simulink model "simul3"  (R2023b)
settings: Solver=ode4  StartTime=0.0  StopTime=600  FixedStep=0.0002  RelTol=1e-3
InitFcn:
  | init3
StopFcn:
  | stop3
values from neighbouring files (symbols this model uses):
  eps_capteur = +0.03    (= 0.03)    [init3.m]
  fs = 5000    [init3.m]
  G_pga = G_pga_vib    (= 10)    [init3.m]
  G_pga_choc = Vref_adc / (plage_g_choc * K_s)    (= 1)    [init3.m]
  G_pga_vib = Vref_adc / (plage_g_vib  * K_s)    (= 10)    [init3.m]
  K_s = 50e-3    (= 0.05)    [init3.m]
  LSB_V = 2 * Vref_adc / 2^n_bits    (= 0.000152587890625)    [init3.m]
  M_dec = 10    [init3.m]
  ordre_aaf = 4    [init3.m]
  tau_IEPE = 1 / (2 * pi * f_c_IEPE)    (= 0.318309886184)    [init3.m]
libraries: dspfdesign x1, simulink x1, dspmlti4 x1
settings Model: Creator=xavie  LastModifiedBy=xavie
settings DataIOCC: ReturnWorkspaceOutputs=off

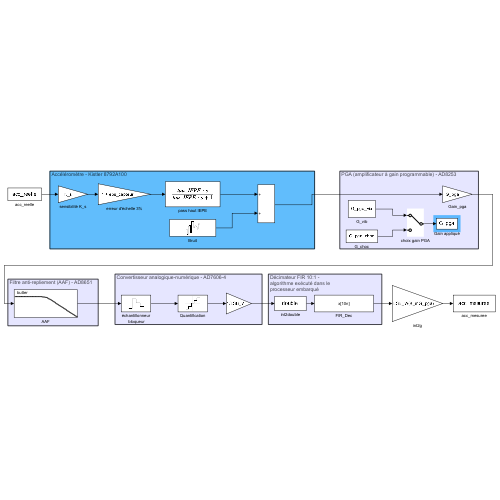
[thumbnail: Simulink's stored preview of the top-level diagram]
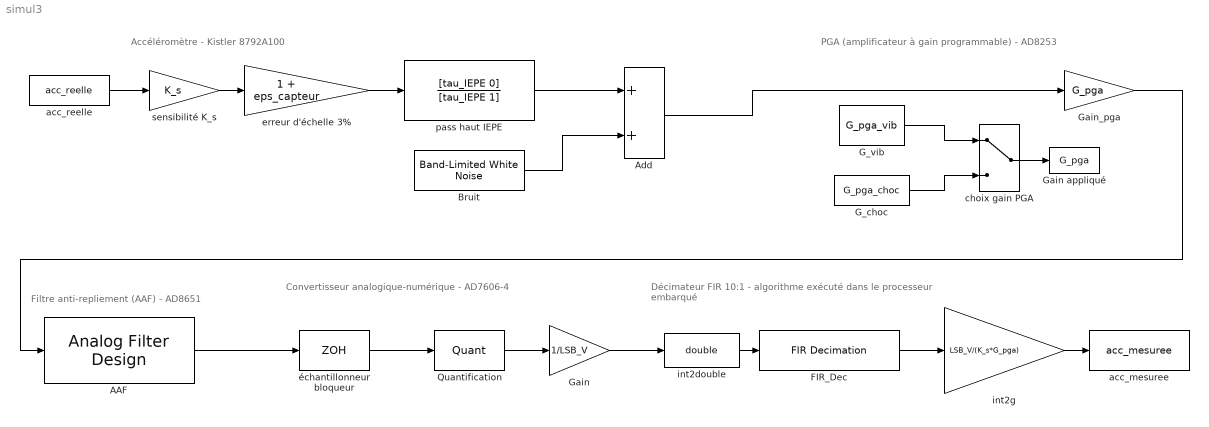
== system simul3 ==
  note: Décimateur FIR 10:1 -
      | algorithme exécuté dans le
      | processeur embarqué
  note: Convertisseur analogique-numérique - AD7606-4
  note: Filtre anti-repliement (AAF) - AD8651
  note: PGA (amplificateur à gain programmable) - AD8253
  note: Accéléromètre - Kistler 8792A100
  AAF : dspfdesign/Analog Filter Design  method=Butterworth  filttype=Lowpass  N=ordre_aaf  Wlo=omega_aaf  Whi=80  Rp=2  Rs=40
  Add : Sum
  Bruit : simulink/Sources/Band-Limited White Noise  Cov=bruit_capteur_power  Ts=0.0002  seed=1234
  FIR_Dec : dspmlti4/FIR Decimation  FilterSource=Auto  h=h_dec  D=M_dec  filtStruct=Direct form  FilterObject=FDECIM  InputProcessing=Columns as channels (frame based)  framing=Allow multirate processing  AllowArbitraryInputLength=off  inputOffset=0  outputBufInitCond=0  roundingMode=Floor  overflowMode=off  firstCoeffDataTypeStr=Inherit: Same word length as input  firstCoeffMin=[]  firstCoeffMax=[]  firstCoeffLastDataTypeStr=Inherit: Same word length as input  outputDataTypeStr=Inherit: Same as accumulator  outputMin=[]  outputMax=[]  outputLastDataTypeStr=Inherit: Same as accumulator
  G_choc : Constant  Value=G_pga_choc
  G_vib : Constant  Value=G_pga_vib
  Gain : Gain  Gain=1/LSB_V  OutDataTypeStr=int16
  Gain appliqué : ToWorkspace  VariableName=G_pga  SampleTime=-1
      settings: MaxDataPoints=1
  Gain_pga : Gain  Gain=G_pga
  Quantification : Quantizer  QuantizationInterval=LSB_V
  acc_mesuree : ToWorkspace  VariableName=acc_mesuree  SampleTime=-1
  acc_reelle : FromWorkspace  VariableName=acc_reelle  SampleTime=-1
  choix gain PGA : ManualSwitch
  erreur d'échelle 3% : Gain  Gain=1 + eps_capteur
  int2double : DataTypeConversion  OutDataTypeStr=double  SaturateOnIntegerOverflow=off  RndMeth=Floor
  int2g : Gain  Gain=LSB_V/(K_s*G_pga)
  pass haut IEPE : TransferFcn  Numerator=[tau_IEPE 0]  Denominator=[tau_IEPE 1]
  sensibilité K_s : Gain  Gain=K_s
  échantillonneur bloqueur : ZeroOrderHold  SampleTime=1/fs
  wires:
  G_vib/1 -> choix gain PGA/1
  G_choc/1 -> choix gain PGA/2
  AAF/1 -> échantillonneur bloqueur/1
  échantillonneur bloqueur/1 -> Quantification/1
  Quantification/1 -> Gain/1
  FIR_Dec/1 -> int2g/1
  int2g/1 -> acc_mesuree/1
  sensibilité K_s/1 -> erreur d'échelle 3%/1
  acc_reelle/1 -> sensibilité K_s/1
  choix gain PGA/1 -> Gain appliqué/1
  Gain_pga/1 -> AAF/1
  Gain/1 -> int2double/1
  int2double/1 -> FIR_Dec/1
  erreur d'échelle 3%/1 -> pass haut IEPE/1
  Add/1 -> Gain_pga/1
  pass haut IEPE/1 -> Add/1
  Bruit/1 -> Add/2
